simulink model "simu"  (R2021b)
settings: Solver=VariableStepAuto  StartTime=0.0  StopTime=10.0  RelTol=1e-3
undefined symbols (not defined in the file or in its folder): DCD, DCM0, DCM1, NCD, NCM0, NCM1
settings Model: Creator=gabri  LastModifiedBy=gabri

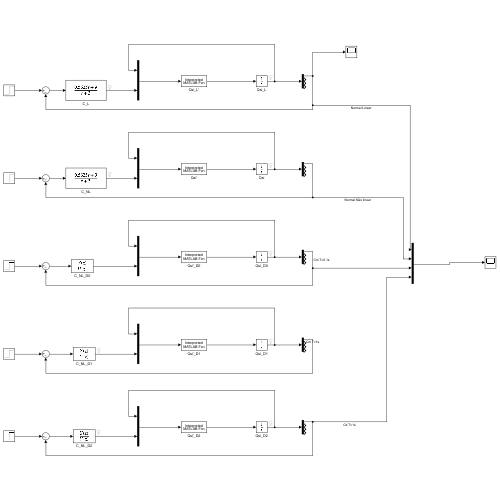
[thumbnail: Simulink's stored preview of the top-level diagram]
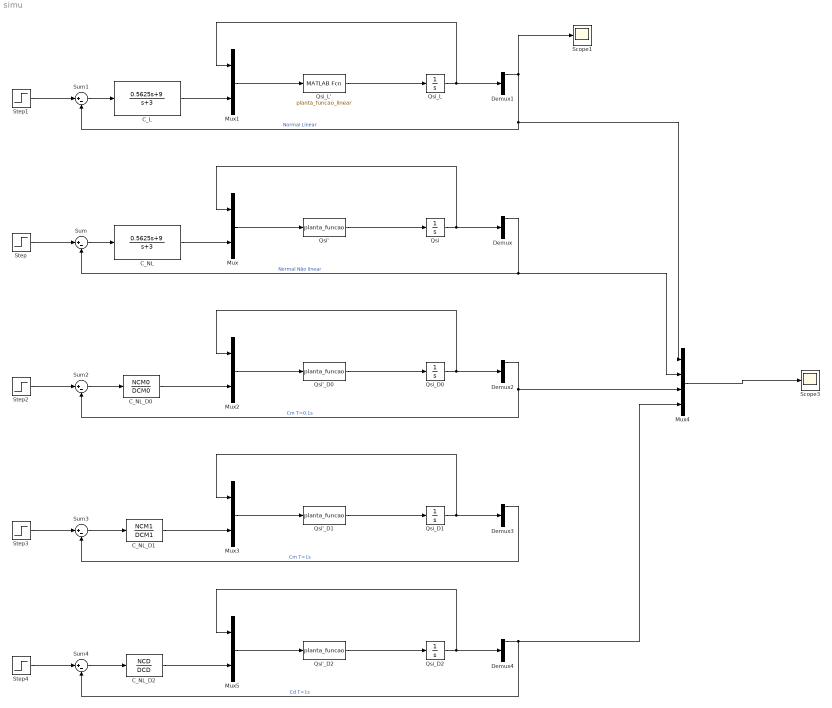
== system simu ==
  C_L : TransferFcn  Numerator=[0.5625 9]  Denominator=[1 3]
  C_NL : TransferFcn  Numerator=[0.5625 9]  Denominator=[1 3]
  C_NL_D0 : DiscreteTransferFcn  Numerator=NCM0  Denominator=DCM0  SampleTime=0.1
  C_NL_D1 : DiscreteTransferFcn  Numerator=NCM1  Denominator=DCM1  SampleTime=1
  C_NL_D2 : DiscreteTransferFcn  Numerator=NCD  Denominator=DCD  SampleTime=1
  Demux{,1..4} (5 alike) : Demux
  Mux{,1..3,5} (5 alike) : Mux  Inputs=2
  Mux4 : Mux
  Qsi : Integrator
  Qsi' : MATLABFcn  MATLABFcn=planta_funcao  OutputDimensions=4
  Qsi'_D0 : MATLABFcn  MATLABFcn=planta_funcao  OutputDimensions=4
  Qsi'_D1 : MATLABFcn  MATLABFcn=planta_funcao  OutputDimensions=4
  Qsi'_D2 : MATLABFcn  MATLABFcn=planta_funcao  OutputDimensions=4
  Qsi_D0 : Integrator
  Qsi_D1 : Integrator
  Qsi_D2 : Integrator
  Qsi_L : Integrator
  Qsi_L' : MATLABFcn  MATLABFcn=planta_funcao_linear  OutputDimensions=4
  Scope1 : Scope
  Scope3 : Scope
  Step{,1..4} (5 alike) : Step  Time=0  After=10  SampleTime=0
  Sum{,1..4} (5 alike) : Sum  Inputs=|+-
  wires:
  C_NL/1 -> Mux/2
  Qsi'/1 -> Qsi/1
  Qsi/1 -> Demux/1, Mux/1
  Mux/1 -> Qsi'/1
  Step/1 -> Sum/1
  Sum/1 -> C_NL/1
  Demux/1 -> Mux4/2, Sum/2  "Normal Não linear"
  Demux1/1 -> Mux4/1, Sum1/2, Scope1/1  "Normal Linear"
  Sum1/1 -> C_L/1
  Qsi_L/1 -> Demux1/1, Mux1/1
  C_L/1 -> Mux1/2
  Step1/1 -> Sum1/1
  Mux1/1 -> Qsi_L'/1
  Qsi_L'/1 -> Qsi_L/1
  Mux2/1 -> Qsi'_D0/1
  Step2/1 -> Sum2/1
  Qsi_D0/1 -> Demux2/1, Mux2/1
  Sum2/1 -> C_NL_D0/1
  Qsi'_D0/1 -> Qsi_D0/1
  Demux2/1 -> Mux4/3, Sum2/2  "Cm T=0.1s"
  Sum3/1 -> C_NL_D1/1
  Qsi_D1/1 -> Demux3/1, Mux3/1
  Qsi'_D1/1 -> Qsi_D1/1
  Demux3/1 -> Sum3/2  "Cm T=1s"
  Mux3/1 -> Qsi'_D1/1
  C_NL_D1/1 -> Mux3/2
  Step3/1 -> Sum3/1
  Mux4/1 -> Scope3/1
  C_NL_D0/1 -> Mux2/2
  Sum4/1 -> C_NL_D2/1
  C_NL_D2/1 -> Mux5/2
  Demux4/1 -> Mux4/4, Sum4/2  "Cd T=1s"
  Mux5/1 -> Qsi'_D2/1
  Step4/1 -> Sum4/1
  Qsi'_D2/1 -> Qsi_D2/1
  Qsi_D2/1 -> Demux4/1, Mux5/1
